simulink model "OneModule"  (R2016a)
settings: Solver=VariableStepAuto  StartTime=0.0  StopTime=0.7  RelTol=1e-3
libraries: fl_lib x8, nesl_utility x6, powerlib_meascontrol x5, pe_lib x4, dspstat3 x1
settings Model: Creator=ugurm  LastModifiedBy=ugurm

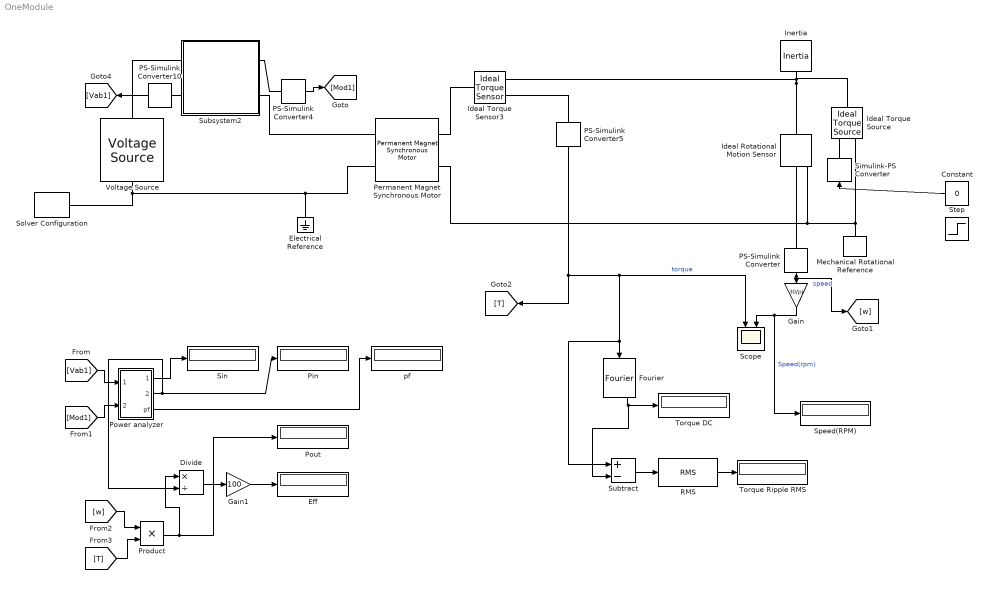
== system OneModule ==
  Constant : Constant  Value=0
  Divide : Product  Inputs=*/
  Eff : Display
  Electrical Reference : fl_lib/Electrical/Electrical Elements/Electrical Reference
  Fourier : powerlib_meascontrol/Measurements/Fourier  Freq=freq  n=0  InInit=[0, 0]  Ts=0
  Gain : Gain  Gain=30/pi
  Gain1 : Gain  Gain=100
  Ideal Rotational Motion Sensor : fl_lib/Mechanical/Mechanical Sensors/Ideal Rotational Motion Sensor  offset=0 rad
  Ideal Torque Sensor3 : fl_lib/Mechanical/Mechanical Sensors/Ideal Torque Sensor
  Ideal Torque Source : fl_lib/Mechanical/Mechanical Sources/Ideal Torque Source
  Inertia : fl_lib/Mechanical/Rotational Elements/Inertia  inertia=10 kg*m^2  w_specify=on  w_priority=High  w=0 rad/s  t_specify=on  t_priority=Low  t=0 N*m
  Mechanical Rotational Reference : fl_lib/Mechanical/Rotational Elements/Mechanical Rotational Reference
  PS-Simulink Converter{,4..5,10} (4 alike) : nesl_utility/PS-Simulink Converter  PhysicalDomain=network_engine_domain  SubClassName=ps_output  LeftPortType=input  RightPortType=output  PseudoPeriodic=off  Frequencies=[]  Unit=1  AffineConversion=off
  Permanent Magnet Synchronous Motor : pe_lib/Machines/Permanent Magnet Rotor/Permanent Magnet Synchronous Motor  nPolePairs=4  pm_flux_linkage=0.192 Wb  stator_param=1  Ld=603.3 uH  Lq=666.8 uH  L0=0 uH  Ls=0.0002 H  Lm=0.00002 H  Ms=0.00002 H  Rs=0.05 Ohm  initial_currents=[0.0, 0.0, 0.0] A  axes_param=2  angular_position0=0 deg  rotor_offset=- pi / 2 rad  shift_3ph=[nan, nan, nan] rad  sqrt2OverSqrt3=nan  oneOverSqrt2=nan  twoPiOver3=nan  Lmin=1e-9 H
  Pin : Display
  Pout : Display
  Power analyzer : Subsystem
  Product : Product
  RMS : dspstat3/RMS  run=off  reset_popup=None  InputProcessing=Columns as channels (frame based)  directionMode=Each column  dimension=1
  Scope : Scope  NumInputPorts=2
  Simulink-PS Converter : nesl_utility/Simulink-PS Converter  PhysicalDomain=network_engine_domain  SubClassName=ps_input  LeftPortType=input  RightPortType=output  PseudoPeriodic=off  Frequencies=[]  NoiseDistribution=none  NoiseParameters=[]  Unit=1  AffineConversion=off  InputFiltering=off  SimscapeFilterOrder=1  InputFilterTimeConstant=0.001  UdotUserProvided=1
  Sin : Display
  Solver Configuration : nesl_utility/Solver Configuration  PhysicalDomain=network_engine_domain  SubClassName=solver  LeftPortType=input  RightPortType=generic  Accelerate=off  Tones=[]  Harmonics=[]  SimulateNoise=off  Profile=off  UseLocalSampling=off  EnableSwitchedLinearOptims=on  FrequencyDomain=off  UseCCode=off  RelTol=0.001  AbsTol=1e-06  MinStep=1e-09  ToWorkspace=off  RevertToSquareIcSolve=off  NumHomotopyIterations=100  PhasorMode=off  PhasorModeNumHarmonics=1  OverrideAbsTol=off  DoDC=off  ResidualTolerance=1e-09  UseLocalSolver=on  LocalSolverChoice=NE_BACKWARD_EULER_ADVANCER  LocalSolverSampleTime=1e-06  DoFixedCost=on  MaxNonlinIter=3  MaxModeIter=2  LinearAlgebra=Sparse  DelaysMemoryBudget=1024  AutomaticFiltering=on  FilteringTimeConstant=0.001
  Speed(RPM) : Display
  Step : Step  Time=0.1  After=100  SampleTime=0
  Subsystem2 : Subsystem
  Subtract : Sum  Inputs=+-
  Torque DC : Display
  Torque Ripple RMS : Display
  Voltage Source : pe_lib/Sources/Voltage Source  vline_rms=sqrt(3) * 220 V  shift=0 deg  freq=freq Hz  harmonic_option=0  harmonic_orders=[5.0, 7.0, 11.0, 13.0]  harmonic_ratios=[0.1, 0.1, 0.1, 0.1]
  pf : Display
  wires:
  PS-Simulink Converter4/1 -> [Mod1]
  Constant/1 -> Simulink-PS Converter/1
  PS-Simulink Converter10/1 -> [Vab1]
  [Vab1] -> Power analyzer/1(In1)
  [Mod1] -> Power analyzer/2(In2)
  Power analyzer/1(Sin) -> Sin/1
  Power analyzer/2(Pin) -> Divide/2, Pin/1
  Power analyzer/3(pf) -> pf/1
  PS-Simulink Converter5/1 -> [T], Subtract/1, Fourier/1, Scope/1  "torque"
  Fourier/1 -> Subtract/2, Torque DC/1
  Subtract/1 -> RMS/1
  RMS/1 -> Torque Ripple RMS/1
  PS-Simulink Converter/1 -> [w], Gain/1  "speed"
  Gain/1 -> Speed(RPM)/1, Scope/2  "Speed(rpm)"
  [w] -> Product/1
  [T] -> Product/2
  Product/1 -> Divide/1, Pout/1
  Divide/1 -> Gain1/1
  Gain1/1 -> Eff/1
  connections:
  Solver Configuration/RConn1 -- Voltage Source/LConn1 -- Electrical Reference/LConn1 -- Permanent Magnet Synchronous Motor/LConn2
  Mechanical Rotational Reference/LConn1 -- Permanent Magnet Synchronous Motor/RConn2 -- Ideal Rotational Motion Sensor/RConn1 -- Ideal Torque Source/RConn2
  Ideal Torque Source/LConn1 -- Ideal Rotational Motion Sensor/LConn1 -- Inertia/LConn1 -- Ideal Torque Sensor3/RConn1
  PS-Simulink Converter10/LConn1 -- Subsystem2/LConn2
  Simulink-PS Converter/RConn1 -- Ideal Torque Source/RConn1
  PS-Simulink Converter/LConn1 -- Ideal Rotational Motion Sensor/RConn2
  Subsystem2/LConn1 -- Voltage Source/RConn1
  PS-Simulink Converter5/LConn1 -- Ideal Torque Sensor3/RConn2
  Subsystem2/RConn2 -- Permanent Magnet Synchronous Motor/LConn1
  PS-Simulink Converter4/LConn1 -- Subsystem2/RConn1
  Ideal Torque Sensor3/LConn1 -- Permanent Magnet Synchronous Motor/RConn1

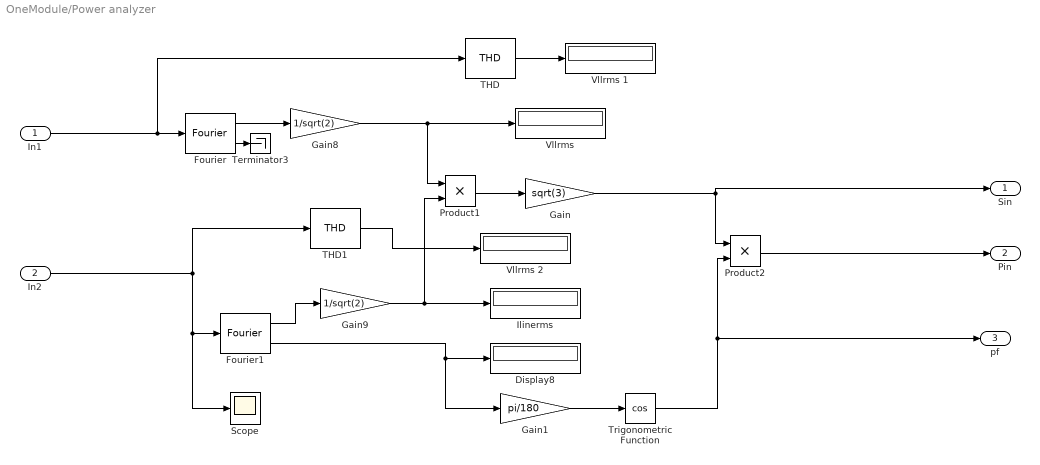
== system OneModule/Power analyzer ==
  In1 : Inport
  In2 : Inport  Port=2
  Display8 : Display
  Fourier : powerlib_meascontrol/Measurements/Fourier  Freq=freq  n=1  InInit=[0, 0]  Ts=0
  Fourier1 : powerlib_meascontrol/Measurements/Fourier  Freq=freq  n=1  InInit=[0, 0]  Ts=0
  Gain : Gain  Gain=sqrt(3)
  Gain1 : Gain  Gain=pi/180
  Gain8 : Gain  Gain=1/sqrt(2)
  Gain9 : Gain  Gain=1/sqrt(2)
  "Ilinerms " : Display
  Product1 : Product
  Product2 : Product
  Scope : Scope
  THD : powerlib_meascontrol/Measurements/THD  Freq=freq  Ts=0
  THD1 : powerlib_meascontrol/Measurements/THD  Freq=freq  Ts=0
  Terminator3 : Terminator
  Trigonometric Function : Trigonometry  Operator=cos
  "Vllrms " : Display
  Vllrms 1 : Display
  Vllrms 2 : Display
  Sin : Outport
  Pin : Outport  Port=2
  pf : Outport  Port=3
  wires:
  Gain8/1 -> Product1/1, "Vllrms "/1
  Gain9/1 -> "Ilinerms "/1, Product1/2
  In2/1 -> Scope/1, Fourier1/1, THD1/1
  Fourier1/1 -> Gain9/1
  In1/1 -> THD/1, Fourier/1
  Fourier/1 -> Gain8/1
  Product1/1 -> Gain/1
  Gain/1 -> Sin/1, Product2/1
  Fourier1/2 -> Gain1/1, Display8/1
  Trigonometric Function/1 -> pf/1, Product2/2
  Gain1/1 -> Trigonometric Function/1
  Product2/1 -> Pin/1
  Fourier/2 -> Terminator3/1
  THD/1 -> Vllrms 1/1
  THD1/1 -> Vllrms 2/1

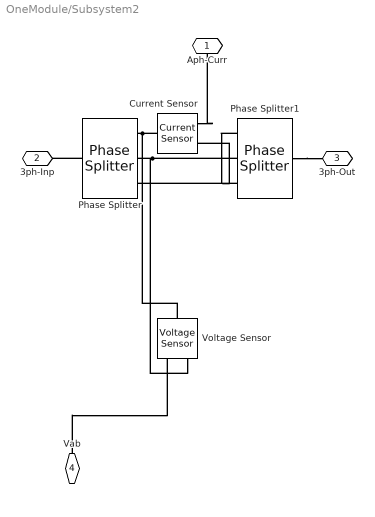
== system OneModule/Subsystem2 ==
  Current Sensor : fl_lib/Electrical/Electrical Sensors/Current Sensor
  Phase Splitter : pe_lib/Connections/Phase Splitter
  Phase Splitter1 : pe_lib/Connections/Phase Splitter
  Voltage Sensor : fl_lib/Electrical/Electrical Sensors/Voltage Sensor
  Aph-Curr : PMIOPort  Port=1  Side=Right
  3ph-Inp : PMIOPort  Port=2  Side=Left
  3ph-Out : PMIOPort  Port=3  Side=Right
  Vab : PMIOPort  Port=4  Side=Left
  connections:
  Phase Splitter1/LConn1 -- 3ph-Out/RConn1
  Phase Splitter/LConn1 -- 3ph-Inp/RConn1
  Phase Splitter1/RConn1 -- Current Sensor/RConn2
  Current Sensor/LConn1 -- Phase Splitter/RConn1 -- Voltage Sensor/LConn1
  Current Sensor/RConn1 -- Aph-Curr/RConn1
  Phase Splitter1/RConn3 -- Phase Splitter/RConn3
  Phase Splitter1/RConn2 -- Voltage Sensor/RConn2 -- Phase Splitter/RConn2
  Vab/RConn1 -- Voltage Sensor/RConn1
